simulink model "Lecture13_StepResponse"  (R2020b)
settings: Solver=VariableStepAuto  StartTime=0.0  StopTime=10.0  RelTol=1e-3
values from neighbouring files (symbols this model uses):
  Gs_den = [1 2 1]    [Lecture13_StepResponse.m]
  Gs_num = [10]    [Lecture13_StepResponse.m]
  Gz_den = Gz_slow.Denominator{1,1}    [Lecture13_StepResponse.m]
  Gz_num = Gz_slow.Numerator{1,1}    [Lecture13_StepResponse.m]
  T_samp = 1./(f_samp)    [Lecture13_StepResponse.m]
settings Model: Creator=sebastian  LastModifiedBy=sebastian

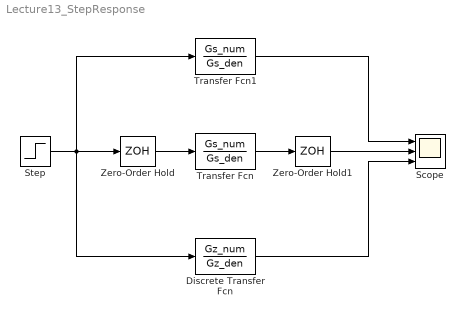
== system Lecture13_StepResponse ==
  Discrete Transfer Fcn : DiscreteTransferFcn  Numerator=Gz_num  Denominator=Gz_den  SampleTime=T_samp
  Scope : Scope  NumInputPorts=3
  Step : Step  SampleTime=0
  Transfer Fcn : TransferFcn  Numerator=Gs_num  Denominator=Gs_den
  Transfer Fcn1 : TransferFcn  Numerator=Gs_num  Denominator=Gs_den
  Zero-Order Hold : ZeroOrderHold  SampleTime=T_samp
  Zero-Order Hold1 : ZeroOrderHold  SampleTime=T_samp
  wires:
  Step/1 -> Discrete Transfer Fcn/1, Transfer Fcn1/1, Zero-Order Hold/1
  Zero-Order Hold/1 -> Transfer Fcn/1
  Transfer Fcn/1 -> Zero-Order Hold1/1
  Zero-Order Hold1/1 -> Scope/2
  Discrete Transfer Fcn/1 -> Scope/3
  Transfer Fcn1/1 -> Scope/1
